simulink model "Electromech"  (R2023b)
settings: Solver=VariableStepAuto  StartTime=0.0  StopTime=10.0  RelTol=1e-3
settings Model: Creator=Nishanth S  LastModifiedBy=Nishanth S

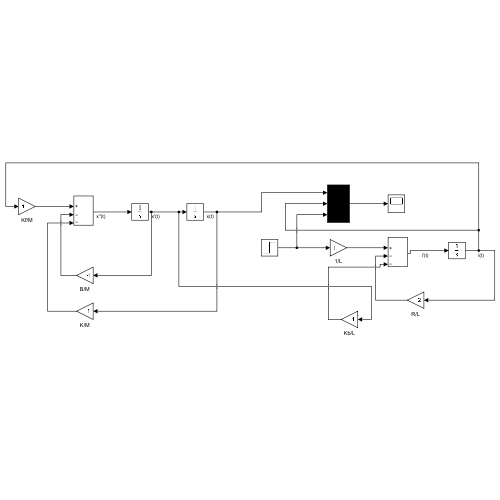
[thumbnail: Simulink's stored preview of the top-level diagram]
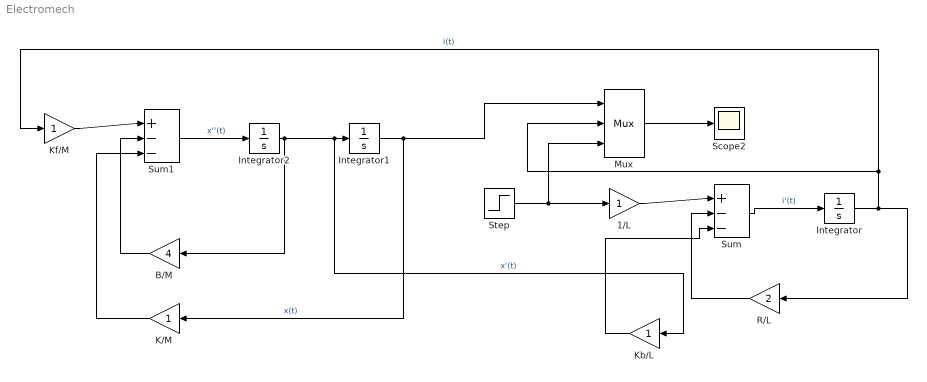
== system Electromech ==
  1/L : Gain
  B/M : Gain  Gain=4
  Integrator : Integrator
  Integrator1 : Integrator
  Integrator2 : Integrator
  K/M : Gain
  Kb/L : Gain
  Kf/M : Gain
  Mux : Mux  Inputs=3
  R/L : Gain  Gain=2
  Scope2 : Scope
  Step : Step  SampleTime=0
  Sum : Sum  Inputs=|+--
  Sum1 : Sum  Inputs=|+--
  wires:
  Step/1 -> 1/L/1, Mux/3
  1/L/1 -> Sum/1
  Sum/1 -> Integrator/1  "i'(t)"
  Integrator/1 -> R/L/1, Mux/2, Kf/M/1  "i(t)"
  R/L/1 -> Sum/2
  Kf/M/1 -> Sum1/1
  Sum1/1 -> Integrator2/1  "x''(t)"
  Integrator2/1 -> B/M/1, Kb/L/1, Integrator1/1  "x'(t)"
  Integrator1/1 -> Mux/1, K/M/1  "x(t)"
  Kb/L/1 -> Sum/3
  B/M/1 -> Sum1/2
  K/M/1 -> Sum1/3
  Mux/1 -> Scope2/1
